simulink model "example1"  (R2024b)
settings: Solver=FixedStepAuto  StartTime=0.0  StopTime=20  FixedStep=0.001  RelTol=1e-3
(part 2 of 3)

== system example1/alpha1 ==
  p/q : Inport
  sumDFj-DFi : Inport  Port=2
  ei1 : Inport  Port=3
  x11 : Inport  Port=4
  Constant : Constant  Value=2
  Gain : Gain  Gain=-1
  Gain1 : Gain  Gain=-0.5
  SAT : Subsystem  Commented=through
  Scope : Scope
  Scope1 : Scope
  Scope2 : Scope
  Sum : Sum  Inputs=|+-
  Sum1 : Sum  Inputs=|++
  Sum2 : Sum  Inputs=|+-
  Sum3 : Sum  Inputs=+++
  "[2]^1_1" : Subsystem
  "[2]^1_2" : Subsystem
  g11 : Subsystem
  alpha1 : Outport
  wires:
  Constant/1 -> Sum/1
  p/q/1 -> "[2]^1_2"/1(p/q), Sum/2
  ei1/1 -> "[2]^1_2"/2(2), "[2]^1_1"/2(2), Gain1/1, Scope/1
  Sum/1 -> "[2]^1_1"/1(In1)
  "[2]^1_1"/1(Out1) -> Sum1/1
  "[2]^1_2"/1(Out1) -> Sum1/2
  Sum1/1 -> Gain/1
  Gain/1 -> Sum3/2
  Sum3/1 -> Sum2/1, Scope2/1
  Gain1/1 -> Sum3/1
  sumDFj-DFi/1 -> Scope1/1, Sum3/3
  g11/1(g11) -> Sum2/2
  x11/1 -> g11/1(x11)
  Sum2/1 -> SAT/1(In1)
  SAT/1(u1) -> alpha1/1

== system example1/alpha2 ==
  p/q : Inport
  sumDFj-DFi : Inport  Port=2
  ei2 : Inport  Port=3
  x21 : Inport  Port=4
  Constant : Constant  Value=2
  Gain : Gain  Gain=-1
  Gain1 : Gain  Gain=-0.5
  Sum : Sum  Inputs=|+-
  Sum1 : Sum  Inputs=|++
  Sum2 : Sum  Inputs=|+-
  Sum3 : Sum  Inputs=+++
  "[2]^1_1" : Subsystem
  "[2]^1_2" : Subsystem
  g21 : Subsystem
  alpha2 : Outport
  wires:
  Constant/1 -> Sum/1
  p/q/1 -> "[2]^1_1"/1(p/q), Sum/2
  ei2/1 -> "[2]^1_1"/2(2), "[2]^1_2"/2(2), Gain1/1
  Sum/1 -> "[2]^1_2"/1(In1)
  "[2]^1_2"/1(Out1) -> Sum1/1
  "[2]^1_1"/1(Out1) -> Sum1/2
  Sum1/1 -> Gain/1
  Gain/1 -> Sum3/2
  Gain1/1 -> Sum3/1
  sumDFj-DFi/1 -> Sum3/3
  Sum3/1 -> Sum2/1
  Sum2/1 -> alpha2/1
  x21/1 -> g21/1(x21)
  g21/1(g21) -> Sum2/2

== system example1/alpha3 ==
  p/q : Inport
  sumDFj-DFi : Inport  Port=2
  ei3 : Inport  Port=3
  x31 : Inport  Port=4
  Constant : Constant  Value=2
  Gain : Gain  Gain=-1
  Gain1 : Gain  Gain=-0.5
  Scope : Scope
  Scope1 : Scope
  Sum : Sum  Inputs=|+-
  Sum1 : Sum  Inputs=|++
  Sum2 : Sum  Inputs=|+-
  Sum3 : Sum  Inputs=+++
  Sum4 : Sum  Inputs=|+-
  "[2]^1_1" : Subsystem
  "[2]^1_2" : Subsystem
  g11 : Subsystem
  alpha3 : Outport
  wires:
  Constant/1 -> Sum/1
  p/q/1 -> Sum/2, "[2]^1_1"/1(p/q)
  ei3/1 -> "[2]^1_1"/2(2), "[2]^1_2"/2(2), Gain1/1
  Sum/1 -> "[2]^1_2"/1(In1)
  "[2]^1_2"/1(Out1) -> Sum1/1
  "[2]^1_1"/1(Out1) -> Sum1/2
  Sum1/1 -> Scope/1, Gain/1
  Gain/1 -> Sum3/2
  Gain1/1 -> Sum3/1
  sumDFj-DFi/1 -> Sum3/3
  Sum3/1 -> Sum2/1
  x31/1 -> g11/1(x11)
  g11/1(g11) -> Scope1/1, Sum2/2
  Sum2/1 -> Sum4/1
  Sum4/1 -> alpha3/1

== system example1/alpha4 ==
  p/q : Inport
  ei4 : Inport  Port=2
  sumDFj-DFi : Inport  Port=3
  x41 : Inport  Port=4
  Constant : Constant  Value=2
  Gain : Gain  Gain=-1
  Gain1 : Gain  Gain=-0.5
  Pow : Math  Operator=pow  SignedPower=on  RndMeth=Zero
  Pow1 : Math  Operator=pow  SignedPower=on  RndMeth=Zero
  Sum : Sum  Inputs=|+-
  Sum1 : Sum  Inputs=|++
  Sum3 : Sum  Inputs=+++
  Sum4 : Sum  Inputs=|+-
  g21 : Subsystem
  alpha4 : Outport
  wires:
  Constant/1 -> Sum/1
  p/q/1 -> Pow1/2, Sum/2
  ei4/1 -> Pow1/1, Gain1/1, Pow/1
  Sum/1 -> Pow/2
  Pow/1 -> Sum1/1
  Pow1/1 -> Sum1/2
  Sum1/1 -> Gain/1
  Gain/1 -> Sum3/2
  Gain1/1 -> Sum3/1
  sumDFj-DFi/1 -> Sum3/3
  Sum3/1 -> Sum4/1
  Sum4/1 -> alpha4/1
  x41/1 -> g21/1(x21)
  g21/1(g21) -> Sum4/2

== system example1/alpha5 ==
  p/q : Inport
  sumDFj-DFi : Inport  Port=2
  ei1 : Inport  Port=3
  x11 : Inport  Port=4
  Constant : Constant  Value=2
  Gain : Gain  Gain=-1
  Gain1 : Gain  Gain=-0.5
  SAT : Subsystem  Commented=through
  Scope : Scope
  Scope1 : Scope
  Scope2 : Scope
  Sum : Sum  Inputs=|+-
  Sum1 : Sum  Inputs=|++
  Sum2 : Sum  Inputs=|+-
  Sum3 : Sum  Inputs=+++
  "[2]^1_1" : Subsystem
  "[2]^1_2" : Subsystem
  g11 : Subsystem
  alpha1 : Outport
  wires:
  Constant/1 -> Sum/1
  p/q/1 -> "[2]^1_2"/1(p/q), Sum/2
  ei1/1 -> "[2]^1_2"/2(2), "[2]^1_1"/2(2), Gain1/1, Scope/1
  Sum/1 -> "[2]^1_1"/1(In1)
  "[2]^1_1"/1(Out1) -> Sum1/1
  "[2]^1_2"/1(Out1) -> Sum1/2
  Sum1/1 -> Gain/1
  Gain/1 -> Sum3/2
  Sum3/1 -> Sum2/1, Scope2/1
  Gain1/1 -> Sum3/1
  sumDFj-DFi/1 -> Scope1/1, Sum3/3
  g11/1(g11) -> Sum2/2
  x11/1 -> g11/1(x11)
  Sum2/1 -> SAT/1(In1)
  SAT/1(u1) -> alpha1/1

== system example1/alpha6 ==
  p/q : Inport
  sumDFj-DFi : Inport  Port=2
  ei2 : Inport  Port=3
  x21 : Inport  Port=4
  Constant : Constant  Value=2
  Gain : Gain  Gain=-1
  Gain1 : Gain  Gain=-0.5
  Sum : Sum  Inputs=|+-
  Sum1 : Sum  Inputs=|++
  Sum2 : Sum  Inputs=|+-
  Sum3 : Sum  Inputs=+++
  "[2]^1_1" : Subsystem
  "[2]^1_2" : Subsystem
  g21 : Subsystem
  alpha2 : Outport
  wires:
  Constant/1 -> Sum/1
  p/q/1 -> "[2]^1_1"/1(p/q), Sum/2
  ei2/1 -> "[2]^1_1"/2(2), "[2]^1_2"/2(2), Gain1/1
  Sum/1 -> "[2]^1_2"/1(In1)
  "[2]^1_2"/1(Out1) -> Sum1/1
  "[2]^1_1"/1(Out1) -> Sum1/2
  Sum1/1 -> Gain/1
  Gain/1 -> Sum3/2
  Gain1/1 -> Sum3/1
  sumDFj-DFi/1 -> Sum3/3
  Sum3/1 -> Sum2/1
  Sum2/1 -> alpha2/1
  x21/1 -> g21/1(x21)
  g21/1(g21) -> Sum2/2

== system example1/alpha7 ==
  p/q : Inport
  sumDFj-DFi : Inport  Port=2
  ei3 : Inport  Port=3
  x31 : Inport  Port=4
  Constant : Constant  Value=2
  Gain : Gain  Gain=-1
  Gain1 : Gain  Gain=-0.5
  Scope : Scope
  Scope1 : Scope
  Sum : Sum  Inputs=|+-
  Sum1 : Sum  Inputs=|++
  Sum2 : Sum  Inputs=|+-
  Sum3 : Sum  Inputs=+++
  Sum4 : Sum  Inputs=|+-
  "[2]^1_1" : Subsystem
  "[2]^1_2" : Subsystem
  g11 : Subsystem
  alpha3 : Outport
  wires:
  Constant/1 -> Sum/1
  p/q/1 -> Sum/2, "[2]^1_1"/1(p/q)
  ei3/1 -> "[2]^1_1"/2(2), "[2]^1_2"/2(2), Gain1/1
  Sum/1 -> "[2]^1_2"/1(In1)
  "[2]^1_2"/1(Out1) -> Sum1/1
  "[2]^1_1"/1(Out1) -> Sum1/2
  Sum1/1 -> Scope/1, Gain/1
  Gain/1 -> Sum3/2
  Gain1/1 -> Sum3/1
  sumDFj-DFi/1 -> Sum3/3
  Sum3/1 -> Sum2/1
  x31/1 -> g11/1(x11)
  g11/1(g11) -> Scope1/1, Sum2/2
  Sum2/1 -> Sum4/1
  Sum4/1 -> alpha3/1

== system example1/alpha8 ==
  p/q : Inport
  ei4 : Inport  Port=2
  sumDFj-DFi : Inport  Port=3
  x41 : Inport  Port=4
  Constant : Constant  Value=2
  Gain : Gain  Gain=-1
  Gain1 : Gain  Gain=-0.5
  Pow : Math  Operator=pow  SignedPower=on  RndMeth=Zero
  Pow1 : Math  Operator=pow  SignedPower=on  RndMeth=Zero
  Sum : Sum  Inputs=|+-
  Sum1 : Sum  Inputs=|++
  Sum3 : Sum  Inputs=+++
  Sum4 : Sum  Inputs=|+-
  g21 : Subsystem
  alpha4 : Outport
  wires:
  Constant/1 -> Sum/1
  p/q/1 -> Pow1/2, Sum/2
  ei4/1 -> Pow1/1, Gain1/1, Pow/1
  Sum/1 -> Pow/2
  Pow/1 -> Sum1/1
  Pow1/1 -> Sum1/2
  Sum1/1 -> Gain/1
  Gain/1 -> Sum3/2
  Gain1/1 -> Sum3/1
  sumDFj-DFi/1 -> Sum3/3
  Sum3/1 -> Sum4/1
  Sum4/1 -> alpha4/1
  x41/1 -> g21/1(x21)
  g21/1(g21) -> Sum4/2

== system example1/j-i_1 ==
  DFi : Inport
  DFi+1 : Inport  Port=2
  DFi-1 : Inport  Port=3
  p/q : Inport  Port=4
  Add : Sum  Inputs=+-
  Add1 : Sum  Inputs=-+
  Add2 : Sum  Inputs=-+
  Sum : Sum  Inputs=|++
  Sum1 : Sum  Inputs=|++
  Sum2 : Sum  Inputs=|++
  "[2]^1_1" : Subsystem
  "[2]^1_2" : Subsystem
  "[2]^1_3" : Subsystem
  "[2]^1_4" : Subsystem
  constant : Constant  Value=2
  j-i : Outport
  wires:
  DFi-1/1 -> Add/1
  DFi/1 -> Add1/1, Add/2
  DFi+1/1 -> Add1/2
  p/q/1 -> "[2]^1_4"/1(In1), "[2]^1_3"/1(p/q), Add2/1
  constant/1 -> Add2/2
  Add/1 -> "[2]^1_3"/2(2), "[2]^1_1"/2(2)
  Add2/1 -> "[2]^1_2"/1(In1), "[2]^1_1"/1(In1)
  Add1/1 -> "[2]^1_4"/2(2), "[2]^1_2"/2(2)
  "[2]^1_1"/1(Out1) -> Sum/1
  "[2]^1_2"/1(Out1) -> Sum/2
  "[2]^1_3"/1(Out1) -> Sum1/1
  "[2]^1_4"/1(Out1) -> Sum1/2
  Sum/1 -> Sum2/1
  Sum1/1 -> Sum2/2
  Sum2/1 -> j-i/1

== system example1/j-i_2 ==
  DFi : Inport
  DFi+1 : Inport  Port=2
  DFi-1 : Inport  Port=3
  p/q : Inport  Port=4
  Add : Sum  Inputs=+-
  Add1 : Sum  Inputs=-+
  Add2 : Sum  Inputs=-+
  Sum : Sum  Inputs=|++
  Sum1 : Sum  Inputs=|++
  Sum2 : Sum  Inputs=|++
  "[2]^1_1" : Subsystem
  "[2]^1_2" : Subsystem
  "[2]^1_3" : Subsystem
  "[2]^1_4" : Subsystem
  constant : Constant  Value=2
  j-i : Outport
  wires:
  DFi-1/1 -> Add/1
  DFi/1 -> Add1/1, Add/2
  DFi+1/1 -> Add1/2
  p/q/1 -> "[2]^1_4"/1(In1), "[2]^1_3"/1(In1), Add2/1
  constant/1 -> Add2/2
  Add/1 -> "[2]^1_3"/2(2), "[2]^1_1"/2(2)
  Add2/1 -> "[2]^1_2"/1(In1), "[2]^1_1"/1(In1)
  Add1/1 -> "[2]^1_4"/2(2), "[2]^1_2"/2(2)
  "[2]^1_1"/1(Out1) -> Sum/1
  "[2]^1_2"/1(Out1) -> Sum/2
  "[2]^1_3"/1(Out1) -> Sum1/1
  "[2]^1_4"/1(Out1) -> Sum1/2
  Sum/1 -> Sum2/1
  Sum1/1 -> Sum2/2
  Sum2/1 -> j-i/1

== system example1/j-i_3 ==
  DFi : Inport
  DFi+1 : Inport  Port=2
  DFi-1 : Inport  Port=3
  p/q : Inport  Port=4
  Add : Sum  Inputs=+-
  Add1 : Sum  Inputs=-+
  Add2 : Sum  Inputs=-+
  Pow{,1..3} (4 alike) : Math  Operator=pow  SignedPower=on  RndMeth=Zero
  Scope : Scope
  Scope1 : Scope
  Sum : Sum  Inputs=|++
  Sum1 : Sum  Inputs=|++
  Sum2 : Sum  Inputs=|++
  constant : Constant  Value=2
  j-i : Outport
  wires:
  DFi-1/1 -> Add/1
  DFi/1 -> Add1/1, Add/2
  DFi+1/1 -> Add1/2
  p/q/1 -> Pow3/2, Pow2/2, Add2/1
  constant/1 -> Add2/2
  Add/1 -> Scope1/1, Pow/1, Pow2/1
  Add2/1 -> Pow1/2, Pow/2
  Add1/1 -> Pow3/1, Pow1/1
  Pow/1 -> Sum/1
  Pow1/1 -> Sum/2
  Pow2/1 -> Sum1/1
  Pow3/1 -> Sum1/2
  Sum/1 -> Scope/1, Sum2/1
  Sum1/1 -> Sum2/2
  Sum2/1 -> j-i/1

== system example1/j-i_4 ==
  DFi : Inport
  DFi+1 : Inport  Port=2
  DFi-1 : Inport  Port=3
  p/q : Inport  Port=4
  Add : Sum  Inputs=+-
  Add1 : Sum  Inputs=-+
  Add2 : Sum  Inputs=-+
  Pow{,1..3} (4 alike) : Math  Operator=pow  SignedPower=on  RndMeth=Zero
  Sum : Sum  Inputs=|++
  Sum1 : Sum  Inputs=|++
  Sum2 : Sum  Inputs=|++
  constant : Constant  Value=2
  j-i : Outport
  wires:
  DFi-1/1 -> Add/1
  DFi/1 -> Add1/1, Add/2
  DFi+1/1 -> Add1/2
  p/q/1 -> Pow3/2, Pow2/2, Add2/1
  constant/1 -> Add2/2
  Add/1 -> Pow2/1, Pow/1
  Add2/1 -> Pow1/2, Pow/2
  Add1/1 -> Pow3/1, Pow1/1
  Pow/1 -> Sum/1
  Pow1/1 -> Sum/2
  Pow2/1 -> Sum1/1
  Pow3/1 -> Sum1/2
  Sum/1 -> Sum2/1
  Sum1/1 -> Sum2/2
  Sum2/1 -> j-i/1

== system example1/j-i_5 ==
  DFi : Inport
  DFi+1 : Inport  Port=2
  DFi-1 : Inport  Port=3
  p/q : Inport  Port=4
  Add : Sum  Inputs=+-
  Add1 : Sum  Inputs=-+
  Add2 : Sum  Inputs=-+
  Gain : Gain
  Sum : Sum  Inputs=|++
  Sum1 : Sum  Inputs=|++
  Sum2 : Sum  Inputs=|++
  "[2]^1_1" : Subsystem
  "[2]^1_2" : Subsystem
  "[2]^1_3" : Subsystem
  "[2]^1_4" : Subsystem
  constant : Constant  Value=2
  j-i : Outport
  wires:
  DFi-1/1 -> Add/1
  DFi/1 -> Add1/1, Add/2
  DFi+1/1 -> Add1/2
  p/q/1 -> "[2]^1_4"/1(In1), "[2]^1_3"/1(p/q), Add2/1
  constant/1 -> Add2/2
  Add/1 -> "[2]^1_3"/2(2), "[2]^1_1"/2(2)
  Add2/1 -> "[2]^1_2"/1(In1), "[2]^1_1"/1(In1)
  Add1/1 -> "[2]^1_4"/2(2), "[2]^1_2"/2(2)
  "[2]^1_1"/1(Out1) -> Sum/1
  "[2]^1_2"/1(Out1) -> Sum/2
  "[2]^1_3"/1(Out1) -> Sum1/1
  "[2]^1_4"/1(Out1) -> Sum1/2
  Sum/1 -> Sum2/1
  Sum1/1 -> Sum2/2
  Sum2/1 -> Gain/1
  Gain/1 -> j-i/1

== system example1/j-i_6 ==
  DFi : Inport
  DFi+1 : Inport  Port=2
  DFi-1 : Inport  Port=3
  p/q : Inport  Port=4
  Add : Sum  Inputs=+-
  Add1 : Sum  Inputs=-+
  Add2 : Sum  Inputs=-+
  Gain : Gain
  Sum : Sum  Inputs=|++
  Sum1 : Sum  Inputs=|++
  Sum2 : Sum  Inputs=|++
  "[2]^1_1" : Subsystem
  "[2]^1_2" : Subsystem
  "[2]^1_3" : Subsystem
  "[2]^1_4" : Subsystem
  constant : Constant  Value=2
  j-i : Outport
  wires:
  DFi-1/1 -> Add/1
  DFi/1 -> Add1/1, Add/2
  DFi+1/1 -> Add1/2
  p/q/1 -> "[2]^1_4"/1(In1), "[2]^1_3"/1(In1), Add2/1
  constant/1 -> Add2/2
  Add/1 -> "[2]^1_3"/2(2), "[2]^1_1"/2(2)
  Add2/1 -> "[2]^1_2"/1(In1), "[2]^1_1"/1(In1)
  Add1/1 -> "[2]^1_4"/2(2), "[2]^1_2"/2(2)
  "[2]^1_1"/1(Out1) -> Sum/1
  "[2]^1_2"/1(Out1) -> Sum/2
  "[2]^1_3"/1(Out1) -> Sum1/1
  "[2]^1_4"/1(Out1) -> Sum1/2
  Sum/1 -> Sum2/1
  Sum1/1 -> Sum2/2
  Gain/1 -> j-i/1
  Sum2/1 -> Gain/1

== system example1/j-i_7 ==
  DFi : Inport
  DFi+1 : Inport  Port=2
  DFi-1 : Inport  Port=3
  p/q : Inport  Port=4
  Add : Sum  Inputs=+-
  Add1 : Sum  Inputs=-+
  Add2 : Sum  Inputs=-+
  Gain : Gain
  Pow{,1..3} (4 alike) : Math  Operator=pow  SignedPower=on  RndMeth=Zero
  Scope : Scope
  Scope1 : Scope
  Sum : Sum  Inputs=|++
  Sum1 : Sum  Inputs=|++
  Sum2 : Sum  Inputs=|++
  constant : Constant  Value=2
  j-i : Outport
  wires:
  DFi-1/1 -> Add/1
  DFi/1 -> Add1/1, Add/2
  DFi+1/1 -> Add1/2
  p/q/1 -> Pow3/2, Pow2/2, Add2/1
  constant/1 -> Add2/2
  Add/1 -> Scope1/1, Pow/1, Pow2/1
  Add2/1 -> Pow1/2, Pow/2
  Add1/1 -> Pow3/1, Pow1/1
  Pow/1 -> Sum/1
  Pow1/1 -> Sum/2
  Pow2/1 -> Sum1/1
  Pow3/1 -> Sum1/2
  Sum/1 -> Scope/1, Sum2/1
  Sum1/1 -> Sum2/2
  Sum2/1 -> Gain/1
  Gain/1 -> j-i/1

== system example1/j-i_8 ==
  DFi : Inport
  DFi+1 : Inport  Port=2
  DFi-1 : Inport  Port=3
  p/q : Inport  Port=4
  Add : Sum  Inputs=+-
  Add1 : Sum  Inputs=-+
  Add2 : Sum  Inputs=-+
  Gain : Gain
  Pow{,1..3} (4 alike) : Math  Operator=pow  SignedPower=on  RndMeth=Zero
  Sum : Sum  Inputs=|++
  Sum1 : Sum  Inputs=|++
  Sum2 : Sum  Inputs=|++
  constant : Constant  Value=2
  j-i : Outport
  wires:
  DFi-1/1 -> Add/1
  DFi/1 -> Add1/1, Add/2
  DFi+1/1 -> Add1/2
  p/q/1 -> Pow3/2, Pow2/2, Add2/1
  constant/1 -> Add2/2
  Add/1 -> Pow2/1, Pow/1
  Add2/1 -> Pow1/2, Pow/2
  Add1/1 -> Pow3/1, Pow1/1
  Pow/1 -> Sum/1
  Pow1/1 -> Sum/2
  Pow2/1 -> Sum1/1
  Pow3/1 -> Sum1/2
  Sum/1 -> Sum2/1
  Sum1/1 -> Sum2/2
  Sum2/1 -> Gain/1
  Gain/1 -> j-i/1

== system example1/ESTIMAT1/[2]^1 ==
  In1 : Inport
  In2 : Inport  Port=2
  Abs : Abs  SaturateOnIntegerOverflow=off
  Pow : Math  Operator=pow  SignedPower=on  RndMeth=Zero
  Product : Product
  Sign : Signum
  Out1 : Outport
  wires:
  Pow/1 -> Product/1
  In2/1 -> Abs/1, Sign/1
  Abs/1 -> Pow/1
  Sign/1 -> Product/2
  Product/1 -> Out1/1
  In1/1 -> Pow/2

== system example1/ESTIMAT1/[2]^2 ==
  beta1 : Inport
  In2 : Inport  Port=2
  Abs : Abs  SaturateOnIntegerOverflow=off
  Pow : Math  Operator=pow  SignedPower=on  RndMeth=Zero
  Product : Product
  Sign : Signum
  Out1 : Outport
  wires:
  Pow/1 -> Product/1
  In2/1 -> Abs/1, Sign/1
  Abs/1 -> Pow/1
  Sign/1 -> Product/2
  Product/1 -> Out1/1
  beta1/1 -> Pow/2

== system example1/ESTIMAT1/[2]^3 ==
  In1 : Inport
  In2 : Inport  Port=2
  Abs : Abs  SaturateOnIntegerOverflow=off
  Pow : Math  Operator=pow  SignedPower=on  RndMeth=Zero
  Product : Product
  Sign : Signum
  Out1 : Outport
  wires:
  Pow/1 -> Product/1
  In2/1 -> Abs/1, Sign/1
  Abs/1 -> Pow/1
  Sign/1 -> Product/2
  Product/1 -> Out1/1
  In1/1 -> Pow/2

== system example1/ESTIMAT1/[2]^4 ==
  beta1 : Inport
  In2 : Inport  Port=2
  Abs : Abs  SaturateOnIntegerOverflow=off
  Pow : Math  Operator=pow  SignedPower=on  RndMeth=Zero
  Product : Product
  Sign : Signum
  Out1 : Outport
  wires:
  Pow/1 -> Product/1
  In2/1 -> Abs/1, Sign/1
  Abs/1 -> Pow/1
  Sign/1 -> Product/2
  Product/1 -> Out1/1
  beta1/1 -> Pow/2

== system example1/ESTIMAT1/[2]^5 ==
  In1 : Inport
  In2 : Inport  Port=2
  Abs : Abs  SaturateOnIntegerOverflow=off
  Pow : Math  Operator=pow  SignedPower=on  RndMeth=Zero
  Product : Product
  Sign : Signum
  Out1 : Outport
  wires:
  Pow/1 -> Product/1
  In2/1 -> Abs/1, Sign/1
  Abs/1 -> Pow/1
  Sign/1 -> Product/2
  Product/1 -> Out1/1
  In1/1 -> Pow/2

== system example1/ESTIMAT1/[2]^6 ==
  beta1 : Inport
  In2 : Inport  Port=2
  Abs : Abs  SaturateOnIntegerOverflow=off
  Pow : Math  Operator=pow  SignedPower=on  RndMeth=Zero
  Product : Product
  Sign : Signum
  Out1 : Outport
  wires:
  Pow/1 -> Product/1
  In2/1 -> Abs/1, Sign/1
  Abs/1 -> Pow/1
  Sign/1 -> Product/2
  Product/1 -> Out1/1
  beta1/1 -> Pow/2

== system example1/ESTIMAT1/g11 ==
  x11 : Inport
  Cos : Trigonometry  Operator=cos
  Sum : Sum  Inputs=|++
  g11 : Outport
  wires:
  Cos/1 -> Sum/1
  Sum/1 -> g11/1
  x11/1 -> Sum/2, Cos/1

== system example1/ESTIMAT1/g12 ==
  x11 : Inport
  x12 : Inport  Port=2
  Cos : Trigonometry  Operator=cos
  Sin : Trigonometry
  Sum : Sum  Inputs=|++
  g12 : Outport
  wires:
  x12/1 -> Sin/1
  x11/1 -> Cos/1
  Cos/1 -> Sum/1
  Sin/1 -> Sum/2
  Sum/1 -> g12/1

== system example1/ESTIMAT2/[2]^1 ==
  In1 : Inport
  In2 : Inport  Port=2
  Abs : Abs  SaturateOnIntegerOverflow=off
  Pow : Math  Operator=pow  SignedPower=on  RndMeth=Zero
  Product : Product
  Sign : Signum
  Out1 : Outport
  wires:
  Pow/1 -> Product/1
  In2/1 -> Abs/1, Sign/1
  Abs/1 -> Pow/1
  Sign/1 -> Product/2
  Product/1 -> Out1/1
  In1/1 -> Pow/2

== system example1/ESTIMAT2/[2]^2 ==
  beta1 : Inport
  In2 : Inport  Port=2
  Abs : Abs  SaturateOnIntegerOverflow=off
  Pow : Math  Operator=pow  SignedPower=on  RndMeth=Zero
  Product : Product
  Sign : Signum
  Out1 : Outport
  wires:
  Pow/1 -> Product/1
  In2/1 -> Abs/1, Sign/1
  Abs/1 -> Pow/1
  Sign/1 -> Product/2
  Product/1 -> Out1/1
  beta1/1 -> Pow/2

== system example1/ESTIMAT2/[2]^3 ==
  In1 : Inport
  In2 : Inport  Port=2
  Abs : Abs  SaturateOnIntegerOverflow=off
  Pow : Math  Operator=pow  SignedPower=on  RndMeth=Zero
  Product : Product
  Sign : Signum
  Out1 : Outport
  wires:
  Pow/1 -> Product/1
  In2/1 -> Abs/1, Sign/1
  Abs/1 -> Pow/1
  Sign/1 -> Product/2
  Product/1 -> Out1/1
  In1/1 -> Pow/2

== system example1/ESTIMAT2/[2]^4 ==
  beta1 : Inport
  In2 : Inport  Port=2
  Abs : Abs  SaturateOnIntegerOverflow=off
  Pow : Math  Operator=pow  SignedPower=on  RndMeth=Zero
  Product : Product
  Sign : Signum
  Out1 : Outport
  wires:
  Pow/1 -> Product/1
  In2/1 -> Abs/1, Sign/1
  Abs/1 -> Pow/1
  Sign/1 -> Product/2
  Product/1 -> Out1/1
  beta1/1 -> Pow/2

== system example1/ESTIMAT2/[2]^5 ==
  In1 : Inport
  In2 : Inport  Port=2
  Abs : Abs  SaturateOnIntegerOverflow=off
  Pow : Math  Operator=pow  SignedPower=on  RndMeth=Zero
  Product : Product
  Sign : Signum
  Out1 : Outport
  wires:
  Pow/1 -> Product/1
  In2/1 -> Abs/1, Sign/1
  Abs/1 -> Pow/1
  Sign/1 -> Product/2
  Product/1 -> Out1/1
  In1/1 -> Pow/2

== system example1/ESTIMAT2/[2]^6 ==
  beta1 : Inport
  In2 : Inport  Port=2
  Abs : Abs  SaturateOnIntegerOverflow=off
  Pow : Math  Operator=pow  SignedPower=on  RndMeth=Zero
  Product : Product
  Sign : Signum
  Out1 : Outport
  wires:
  Pow/1 -> Product/1
  In2/1 -> Abs/1, Sign/1
  Abs/1 -> Pow/1
  Sign/1 -> Product/2
  Product/1 -> Out1/1
  beta1/1 -> Pow/2

== system example1/ESTIMAT2/g21 ==
  x21 : Inport
  Cos : Trigonometry  Operator=cos
  Product : Product
  Sin : Trigonometry
  Sum : Sum  Inputs=|++
  g21 : Outport
  wires:
  x21/1 -> Cos/1, Sin/1, Sum/1
  Sum/1 -> g21/1
  Sin/1 -> Product/1
  Cos/1 -> Product/2
  Product/1 -> Sum/2

== system example1/ESTIMAT2/g22 ==
  x21 : Inport
  x22 : Inport  Port=2
  Sin : Trigonometry
  Sum : Sum  Inputs=|++
  Sum1 : Sum  Inputs=|++
  g22 : Outport
  wires:
  x22/1 -> Sum/2, Sum1/2
  Sum/1 -> g22/1
  x21/1 -> Sum1/1
  Sum1/1 -> Sin/1
  Sin/1 -> Sum/1

== system example1/ESTIMAT3/[2]^1 ==
  In1 : Inport
  In2 : Inport  Port=2
  Abs : Abs  SaturateOnIntegerOverflow=off
  Pow : Math  Operator=pow  SignedPower=on  RndMeth=Zero
  Product : Product
  Sign : Signum
  Out1 : Outport
  wires:
  Pow/1 -> Product/1
  In2/1 -> Abs/1, Sign/1
  Abs/1 -> Pow/1
  Sign/1 -> Product/2
  Product/1 -> Out1/1
  In1/1 -> Pow/2

== system example1/ESTIMAT3/[2]^2 ==
  beta1 : Inport
  In2 : Inport  Port=2
  Abs : Abs  SaturateOnIntegerOverflow=off
  Pow : Math  Operator=pow  SignedPower=on  RndMeth=Zero
  Product : Product
  Sign : Signum
  Out1 : Outport
  wires:
  Pow/1 -> Product/1
  In2/1 -> Abs/1, Sign/1
  Abs/1 -> Pow/1
  Sign/1 -> Product/2
  Product/1 -> Out1/1
  beta1/1 -> Pow/2

== system example1/ESTIMAT3/[2]^3 ==
  In1 : Inport
  In2 : Inport  Port=2
  Abs : Abs  SaturateOnIntegerOverflow=off
  Pow : Math  Operator=pow  SignedPower=on  RndMeth=Zero
  Product : Product
  Sign : Signum
  Out1 : Outport
  wires:
  Pow/1 -> Product/1
  In2/1 -> Abs/1, Sign/1
  Abs/1 -> Pow/1
  Sign/1 -> Product/2
  Product/1 -> Out1/1
  In1/1 -> Pow/2

== system example1/ESTIMAT3/[2]^4 ==
  beta1 : Inport
  In2 : Inport  Port=2
  Abs : Abs  SaturateOnIntegerOverflow=off
  Pow : Math  Operator=pow  SignedPower=on  RndMeth=Zero
  Product : Product
  Sign : Signum
  Out1 : Outport
  wires:
  Pow/1 -> Product/1
  In2/1 -> Abs/1, Sign/1
  Abs/1 -> Pow/1
  Sign/1 -> Product/2
  Product/1 -> Out1/1
  beta1/1 -> Pow/2

== system example1/ESTIMAT3/[2]^5 ==
  In1 : Inport
  In2 : Inport  Port=2
  Abs : Abs  SaturateOnIntegerOverflow=off
  Pow : Math  Operator=pow  SignedPower=on  RndMeth=Zero
  Product : Product
  Sign : Signum
  Out1 : Outport
  wires:
  Pow/1 -> Product/1
  In2/1 -> Abs/1, Sign/1
  Abs/1 -> Pow/1
  Sign/1 -> Product/2
  Product/1 -> Out1/1
  In1/1 -> Pow/2

== system example1/ESTIMAT3/[2]^6 ==
  beta1 : Inport
  In2 : Inport  Port=2
  Abs : Abs  SaturateOnIntegerOverflow=off
  Pow : Math  Operator=pow  SignedPower=on  RndMeth=Zero
  Product : Product
  Sign : Signum
  Out1 : Outport
  wires:
  Pow/1 -> Product/1
  In2/1 -> Abs/1, Sign/1
  Abs/1 -> Pow/1
  Sign/1 -> Product/2
  Product/1 -> Out1/1
  beta1/1 -> Pow/2

== system example1/ESTIMAT3/g11 ==
  x11 : Inport
  Sin : Trigonometry
  g11 : Outport
  wires:
  Sin/1 -> g11/1
  x11/1 -> Sin/1

== system example1/ESTIMAT3/g12 ==
  x11 : Inport
  x12 : Inport  Port=2
  Add : Sum  Inputs=3
  Cos : Trigonometry  Operator=cos
  Product : Product
  Sin : Trigonometry
  Sin1 : Trigonometry
  g12 : Outport
  wires:
  x12/1 -> Product/2, Sin/1
  Sin/1 -> Add/2
  Add/1 -> g12/1
  x11/1 -> Product/1, Cos/1
  Cos/1 -> Add/1
  Product/1 -> Sin1/1

== system example1/ESTIMAT4/[2]^1 ==
  In1 : Inport
  In2 : Inport  Port=2
  Abs : Abs  SaturateOnIntegerOverflow=off
  Pow : Math  Operator=pow  SignedPower=on  RndMeth=Zero
  Product : Product
  Sign : Signum
  Out1 : Outport
  wires:
  Pow/1 -> Product/1
  In2/1 -> Abs/1, Sign/1
  Abs/1 -> Pow/1
  Sign/1 -> Product/2
  Product/1 -> Out1/1
  In1/1 -> Pow/2

== system example1/ESTIMAT4/[2]^2 ==
  beta1 : Inport
  In2 : Inport  Port=2
  Abs : Abs  SaturateOnIntegerOverflow=off
  Pow : Math  Operator=pow  SignedPower=on  RndMeth=Zero
  Product : Product
  Sign : Signum
  Out1 : Outport
  wires:
  Pow/1 -> Product/1
  In2/1 -> Abs/1, Sign/1
  Abs/1 -> Pow/1
  Sign/1 -> Product/2
  Product/1 -> Out1/1
  beta1/1 -> Pow/2

== system example1/ESTIMAT4/[2]^3 ==
  In1 : Inport
  In2 : Inport  Port=2
  Abs : Abs  SaturateOnIntegerOverflow=off
  Pow : Math  Operator=pow  SignedPower=on  RndMeth=Zero
  Product : Product
  Sign : Signum
  Out1 : Outport
  wires:
  Pow/1 -> Product/1
  In2/1 -> Abs/1, Sign/1
  Abs/1 -> Pow/1
  Sign/1 -> Product/2
  Product/1 -> Out1/1
  In1/1 -> Pow/2

== system example1/ESTIMAT4/[2]^4 ==
  beta1 : Inport
  In2 : Inport  Port=2
  Abs : Abs  SaturateOnIntegerOverflow=off
  Pow : Math  Operator=pow  SignedPower=on  RndMeth=Zero
  Product : Product
  Sign : Signum
  Out1 : Outport
  wires:
  Pow/1 -> Product/1
  In2/1 -> Abs/1, Sign/1
  Abs/1 -> Pow/1
  Sign/1 -> Product/2
  Product/1 -> Out1/1
  beta1/1 -> Pow/2

== system example1/ESTIMAT4/[2]^5 ==
  In1 : Inport
  In2 : Inport  Port=2
  Abs : Abs  SaturateOnIntegerOverflow=off
  Pow : Math  Operator=pow  SignedPower=on  RndMeth=Zero
  Product : Product
  Sign : Signum
  Out1 : Outport
  wires:
  Pow/1 -> Product/1
  In2/1 -> Abs/1, Sign/1
  Abs/1 -> Pow/1
  Sign/1 -> Product/2
  Product/1 -> Out1/1
  In1/1 -> Pow/2

== system example1/ESTIMAT4/[2]^6 ==
  beta1 : Inport
  In2 : Inport  Port=2
  Abs : Abs  SaturateOnIntegerOverflow=off
  Pow : Math  Operator=pow  SignedPower=on  RndMeth=Zero
  Product : Product
  Sign : Signum
  Out1 : Outport
  wires:
  Pow/1 -> Product/1
  In2/1 -> Abs/1, Sign/1
  Abs/1 -> Pow/1
  Sign/1 -> Product/2
  Product/1 -> Out1/1
  beta1/1 -> Pow/2

== system example1/ESTIMAT4/g21 ==
  x21 : Inport
  Cos : Trigonometry  Operator=cos
  Product : Product
  Product1 : Product
  Sin : Trigonometry
  g21 : Outport
  wires:
  x21/1 -> Cos/1, Sin/1
  Sin/1 -> Product/1
  Product/1 -> g21/1
  Cos/1 -> Product1/1, Product1/2
  Product1/1 -> Product/2

== system example1/ESTIMAT4/g22 ==
  x21 : Inport
  x22 : Inport  Port=2
  Constant : Constant  Value=4/5
  Sin : Trigonometry
  Sum : Sum  Inputs=|++
  Sum1 : Sum  Inputs=|++
  "[2]^1_1" : Subsystem
  g22 : Outport
  wires:
  x22/1 -> Sum1/2, "[2]^1_1"/2(2)
  Constant/1 -> "[2]^1_1"/1(In1)
  "[2]^1_1"/1(Out1) -> Sum/2
  Sum/1 -> g22/1
  x21/1 -> Sum1/1
  Sum1/1 -> Sin/1
  Sin/1 -> Sum/1

== system example1/ESTIMAT5/[2]^1 ==
  In1 : Inport
  In2 : Inport  Port=2
  Abs : Abs  SaturateOnIntegerOverflow=off
  Pow : Math  Operator=pow  SignedPower=on  RndMeth=Zero
  Product : Product
  Sign : Signum
  Out1 : Outport
  wires:
  Pow/1 -> Product/1
  In2/1 -> Abs/1, Sign/1
  Abs/1 -> Pow/1
  Sign/1 -> Product/2
  Product/1 -> Out1/1
  In1/1 -> Pow/2

== system example1/ESTIMAT5/[2]^2 ==
  beta1 : Inport
  In2 : Inport  Port=2
  Abs : Abs  SaturateOnIntegerOverflow=off
  Pow : Math  Operator=pow  SignedPower=on  RndMeth=Zero
  Product : Product
  Sign : Signum
  Out1 : Outport
  wires:
  Pow/1 -> Product/1
  In2/1 -> Abs/1, Sign/1
  Abs/1 -> Pow/1
  Sign/1 -> Product/2
  Product/1 -> Out1/1
  beta1/1 -> Pow/2

== system example1/ESTIMAT5/[2]^3 ==
  In1 : Inport
  In2 : Inport  Port=2
  Abs : Abs  SaturateOnIntegerOverflow=off
  Pow : Math  Operator=pow  SignedPower=on  RndMeth=Zero
  Product : Product
  Sign : Signum
  Out1 : Outport
  wires:
  Pow/1 -> Product/1
  In2/1 -> Abs/1, Sign/1
  Abs/1 -> Pow/1
  Sign/1 -> Product/2
  Product/1 -> Out1/1
  In1/1 -> Pow/2

== system example1/ESTIMAT5/[2]^4 ==
  beta1 : Inport
  In2 : Inport  Port=2
  Abs : Abs  SaturateOnIntegerOverflow=off
  Pow : Math  Operator=pow  SignedPower=on  RndMeth=Zero
  Product : Product
  Sign : Signum
  Out1 : Outport
  wires:
  Pow/1 -> Product/1
  In2/1 -> Abs/1, Sign/1
  Abs/1 -> Pow/1
  Sign/1 -> Product/2
  Product/1 -> Out1/1
  beta1/1 -> Pow/2

== system example1/ESTIMAT5/[2]^5 ==
  In1 : Inport
  In2 : Inport  Port=2
  Abs : Abs  SaturateOnIntegerOverflow=off
  Pow : Math  Operator=pow  SignedPower=on  RndMeth=Zero
  Product : Product
  Sign : Signum
  Out1 : Outport
  wires:
  Pow/1 -> Product/1
  In2/1 -> Abs/1, Sign/1
  Abs/1 -> Pow/1
  Sign/1 -> Product/2
  Product/1 -> Out1/1
  In1/1 -> Pow/2

== system example1/ESTIMAT5/[2]^6 ==
  beta1 : Inport
  In2 : Inport  Port=2
  Abs : Abs  SaturateOnIntegerOverflow=off
  Pow : Math  Operator=pow  SignedPower=on  RndMeth=Zero
  Product : Product
  Sign : Signum
  Out1 : Outport
  wires:
  Pow/1 -> Product/1
  In2/1 -> Abs/1, Sign/1
  Abs/1 -> Pow/1
  Sign/1 -> Product/2
  Product/1 -> Out1/1
  beta1/1 -> Pow/2

== system example1/ESTIMAT5/g21 ==
  x21 : Inport
  Cos : Trigonometry  Operator=cos
  Product : Product
  Sin : Trigonometry  Operator=cos
  Sum : Sum  Inputs=|++
  g21 : Outport
  wires:
  x21/1 -> Sum/1, Sin/1, Cos/1
  Sum/1 -> g21/1
  Sin/1 -> Product/1
  Cos/1 -> Product/2
  Product/1 -> Sum/2

== system example1/ESTIMAT5/g22 ==
  x21 : Inport
  x22 : Inport  Port=2
  Gain : Gain  Gain=-2
  Sin : Trigonometry
  Sum : Sum  Inputs=|++
  Sum1 : Sum  Inputs=|++
  g22 : Outport
  wires:
  x22/1 -> Sum/2, Sum1/2
  Sum/1 -> g22/1
  x21/1 -> Gain/1
  Sum1/1 -> Sin/1
  Sin/1 -> Sum/1
  Gain/1 -> Sum1/1

== system example1/ESTIMAT6/[2]^1 ==
  In1 : Inport
  In2 : Inport  Port=2
  Abs : Abs  SaturateOnIntegerOverflow=off
  Pow : Math  Operator=pow  SignedPower=on  RndMeth=Zero
  Product : Product
  Sign : Signum
  Out1 : Outport
  wires:
  Pow/1 -> Product/1
  In2/1 -> Abs/1, Sign/1
  Abs/1 -> Pow/1
  Sign/1 -> Product/2
  Product/1 -> Out1/1
  In1/1 -> Pow/2

== system example1/ESTIMAT6/[2]^2 ==
  beta1 : Inport
  In2 : Inport  Port=2
  Abs : Abs  SaturateOnIntegerOverflow=off
  Pow : Math  Operator=pow  SignedPower=on  RndMeth=Zero
  Product : Product
  Sign : Signum
  Out1 : Outport
  wires:
  Pow/1 -> Product/1
  In2/1 -> Abs/1, Sign/1
  Abs/1 -> Pow/1
  Sign/1 -> Product/2
  Product/1 -> Out1/1
  beta1/1 -> Pow/2

== system example1/ESTIMAT6/[2]^3 ==
  In1 : Inport
  In2 : Inport  Port=2
  Abs : Abs  SaturateOnIntegerOverflow=off
  Pow : Math  Operator=pow  SignedPower=on  RndMeth=Zero
  Product : Product
  Sign : Signum
  Out1 : Outport
  wires:
  Pow/1 -> Product/1
  In2/1 -> Abs/1, Sign/1
  Abs/1 -> Pow/1
  Sign/1 -> Product/2
  Product/1 -> Out1/1
  In1/1 -> Pow/2

== system example1/ESTIMAT6/[2]^4 ==
  beta1 : Inport
  In2 : Inport  Port=2
  Abs : Abs  SaturateOnIntegerOverflow=off
  Pow : Math  Operator=pow  SignedPower=on  RndMeth=Zero
  Product : Product
  Sign : Signum
  Out1 : Outport
  wires:
  Pow/1 -> Product/1
  In2/1 -> Abs/1, Sign/1
  Abs/1 -> Pow/1
  Sign/1 -> Product/2
  Product/1 -> Out1/1
  beta1/1 -> Pow/2

== system example1/ESTIMAT6/[2]^5 ==
  In1 : Inport
  In2 : Inport  Port=2
  Abs : Abs  SaturateOnIntegerOverflow=off
  Pow : Math  Operator=pow  SignedPower=on  RndMeth=Zero
  Product : Product
  Sign : Signum
  Out1 : Outport
  wires:
  Pow/1 -> Product/1
  In2/1 -> Abs/1, Sign/1
  Abs/1 -> Pow/1
  Sign/1 -> Product/2
  Product/1 -> Out1/1
  In1/1 -> Pow/2

== system example1/ESTIMAT6/[2]^6 ==
  beta1 : Inport
  In2 : Inport  Port=2
  Abs : Abs  SaturateOnIntegerOverflow=off
  Pow : Math  Operator=pow  SignedPower=on  RndMeth=Zero
  Product : Product
  Sign : Signum
  Out1 : Outport
  wires:
  Pow/1 -> Product/1
  In2/1 -> Abs/1, Sign/1
  Abs/1 -> Pow/1
  Sign/1 -> Product/2
  Product/1 -> Out1/1
  beta1/1 -> Pow/2

== system example1/ESTIMAT6/g11 ==
  x11 : Inport
  Sin : Trigonometry  Operator=cos
  g11 : Outport
  wires:
  Sin/1 -> g11/1
  x11/1 -> Sin/1

== system example1/ESTIMAT6/g12 ==
  x11 : Inport
  x12 : Inport  Port=2
  Add : Sum  Inputs=3
  Cos : Trigonometry  Operator=cos
  Gain : Gain  Gain=0.01
  Product : Product
  Sin : Trigonometry
  Sin1 : Trigonometry
  g12 : Outport
  wires:
  x12/1 -> Product/2, Sin/1
  Add/1 -> g12/1
  x11/1 -> Product/1, Cos/1
  Cos/1 -> Add/1
  Product/1 -> Gain/1
  Gain/1 -> Sin1/1
  Sin1/1 -> Add/3
  Sin/1 -> Add/2

== system example1/ESTIMAT7/[2]^1 ==
  In1 : Inport
  In2 : Inport  Port=2
  Abs : Abs  SaturateOnIntegerOverflow=off
  Pow : Math  Operator=pow  SignedPower=on  RndMeth=Zero
  Product : Product
  Sign : Signum
  Out1 : Outport
  wires:
  Pow/1 -> Product/1
  In2/1 -> Abs/1, Sign/1
  Abs/1 -> Pow/1
  Sign/1 -> Product/2
  Product/1 -> Out1/1
  In1/1 -> Pow/2

== system example1/ESTIMAT7/[2]^2 ==
  beta1 : Inport
  In2 : Inport  Port=2
  Abs : Abs  SaturateOnIntegerOverflow=off
  Pow : Math  Operator=pow  SignedPower=on  RndMeth=Zero
  Product : Product
  Sign : Signum
  Out1 : Outport
  wires:
  Pow/1 -> Product/1
  In2/1 -> Abs/1, Sign/1
  Abs/1 -> Pow/1
  Sign/1 -> Product/2
  Product/1 -> Out1/1
  beta1/1 -> Pow/2

== system example1/ESTIMAT7/[2]^3 ==
  In1 : Inport
  In2 : Inport  Port=2
  Abs : Abs  SaturateOnIntegerOverflow=off
  Pow : Math  Operator=pow  SignedPower=on  RndMeth=Zero
  Product : Product
  Sign : Signum
  Out1 : Outport
  wires:
  Pow/1 -> Product/1
  In2/1 -> Abs/1, Sign/1
  Abs/1 -> Pow/1
  Sign/1 -> Product/2
  Product/1 -> Out1/1
  In1/1 -> Pow/2

== system example1/ESTIMAT7/[2]^4 ==
  beta1 : Inport
  In2 : Inport  Port=2
  Abs : Abs  SaturateOnIntegerOverflow=off
  Pow : Math  Operator=pow  SignedPower=on  RndMeth=Zero
  Product : Product
  Sign : Signum
  Out1 : Outport
  wires:
  Pow/1 -> Product/1
  In2/1 -> Abs/1, Sign/1
  Abs/1 -> Pow/1
  Sign/1 -> Product/2
  Product/1 -> Out1/1
  beta1/1 -> Pow/2

== system example1/ESTIMAT7/[2]^5 ==
  In1 : Inport
  In2 : Inport  Port=2
  Abs : Abs  SaturateOnIntegerOverflow=off
  Pow : Math  Operator=pow  SignedPower=on  RndMeth=Zero
  Product : Product
  Sign : Signum
  Out1 : Outport
  wires:
  Pow/1 -> Product/1
  In2/1 -> Abs/1, Sign/1
  Abs/1 -> Pow/1
  Sign/1 -> Product/2
  Product/1 -> Out1/1
  In1/1 -> Pow/2

== system example1/ESTIMAT7/[2]^6 ==
  beta1 : Inport
  In2 : Inport  Port=2
  Abs : Abs  SaturateOnIntegerOverflow=off
  Pow : Math  Operator=pow  SignedPower=on  RndMeth=Zero
  Product : Product
  Sign : Signum
  Out1 : Outport
  wires:
  Pow/1 -> Product/1
  In2/1 -> Abs/1, Sign/1
  Abs/1 -> Pow/1
  Sign/1 -> Product/2
  Product/1 -> Out1/1
  beta1/1 -> Pow/2

== system example1/ESTIMAT7/g21 ==
  x21 : Inport
  Cos : Trigonometry  Operator=cos
  Product : Product
  Sin : Trigonometry
  g21 : Outport
  wires:
  x21/1 -> Cos/1, Sin/1
  Sin/1 -> Product/1
  Product/1 -> g21/1
  Cos/1 -> Product/2

== system example1/ESTIMAT7/g22 ==
  x21 : Inport
  x22 : Inport  Port=2
  Constant : Constant  Value=4/5
  Sin : Trigonometry
  Sum : Sum  Inputs=|++
  Sum1 : Sum  Inputs=|++
  "[2]^1_1" : Subsystem
  g22 : Outport
  wires:
  x22/1 -> "[2]^1_1"/2(2)
  Constant/1 -> "[2]^1_1"/1(In1)
  "[2]^1_1"/1(Out1) -> Sum/2
  Sum/1 -> g22/1
  x21/1 -> Sum1/1
  Sum1/1 -> Sin/1
  Sin/1 -> Sum/1

== system example1/ESTIMAT9/[2]^1 ==
  In1 : Inport
  In2 : Inport  Port=2
  Abs : Abs  SaturateOnIntegerOverflow=off
  Pow : Math  Operator=pow  SignedPower=on  RndMeth=Zero
  Product : Product
  Sign : Signum
  Out1 : Outport
  wires:
  Pow/1 -> Product/1
  In2/1 -> Abs/1, Sign/1
  Abs/1 -> Pow/1
  Sign/1 -> Product/2
  Product/1 -> Out1/1
  In1/1 -> Pow/2

== system example1/ESTIMAT9/[2]^2 ==
  beta1 : Inport
  In2 : Inport  Port=2
  Abs : Abs  SaturateOnIntegerOverflow=off
  Pow : Math  Operator=pow  SignedPower=on  RndMeth=Zero
  Product : Product
  Sign : Signum
  Out1 : Outport
  wires:
  Pow/1 -> Product/1
  In2/1 -> Abs/1, Sign/1
  Abs/1 -> Pow/1
  Sign/1 -> Product/2
  Product/1 -> Out1/1
  beta1/1 -> Pow/2

== system example1/ESTIMAT9/[2]^3 ==
  In1 : Inport
  In2 : Inport  Port=2
  Abs : Abs  SaturateOnIntegerOverflow=off
  Pow : Math  Operator=pow  SignedPower=on  RndMeth=Zero
  Product : Product
  Sign : Signum
  Out1 : Outport
  wires:
  Pow/1 -> Product/1
  In2/1 -> Abs/1, Sign/1
  Abs/1 -> Pow/1
  Sign/1 -> Product/2
  Product/1 -> Out1/1
  In1/1 -> Pow/2

== system example1/ESTIMAT9/[2]^4 ==
  beta1 : Inport
  In2 : Inport  Port=2
  Abs : Abs  SaturateOnIntegerOverflow=off
  Pow : Math  Operator=pow  SignedPower=on  RndMeth=Zero
  Product : Product
  Sign : Signum
  Out1 : Outport
  wires:
  Pow/1 -> Product/1
  In2/1 -> Abs/1, Sign/1
  Abs/1 -> Pow/1
  Sign/1 -> Product/2
  Product/1 -> Out1/1
  beta1/1 -> Pow/2

== system example1/ESTIMAT9/[2]^5 ==
  In1 : Inport
  In2 : Inport  Port=2
  Abs : Abs  SaturateOnIntegerOverflow=off
  Pow : Math  Operator=pow  SignedPower=on  RndMeth=Zero
  Product : Product
  Sign : Signum
  Out1 : Outport
  wires:
  Pow/1 -> Product/1
  In2/1 -> Abs/1, Sign/1
  Abs/1 -> Pow/1
  Sign/1 -> Product/2
  Product/1 -> Out1/1
  In1/1 -> Pow/2

== system example1/ESTIMAT9/[2]^6 ==
  beta1 : Inport
  In2 : Inport  Port=2
  Abs : Abs  SaturateOnIntegerOverflow=off
  Pow : Math  Operator=pow  SignedPower=on  RndMeth=Zero
  Product : Product
  Sign : Signum
  Out1 : Outport
  wires:
  Pow/1 -> Product/1
  In2/1 -> Abs/1, Sign/1
  Abs/1 -> Pow/1
  Sign/1 -> Product/2
  Product/1 -> Out1/1
  beta1/1 -> Pow/2

== system example1/ESTIMAT9/g1 ==
  x11 : Inport
  x12 : Inport  Port=2
  Cos : Trigonometry
  Sin : Trigonometry  Operator=cos
  Sum : Sum  Inputs=|++
  g12 : Outport
  wires:
  x12/1 -> Sin/1
  x11/1 -> Cos/1
  Cos/1 -> Sum/1
  Sin/1 -> Sum/2
  Sum/1 -> g12/1

== system example1/ESTIMAT9/g11 ==
  x11 : Inport
  Cos : Trigonometry
  Sum : Sum  Inputs=|++
  g11 : Outport
  wires:
  Cos/1 -> Sum/1
  Sum/1 -> g11/1
  x11/1 -> Sum/2, Cos/1

== system example1/SYSTEM1/f1 ==
  t : Inport
  x2 : Inport  Port=2
  x1 : Inport  Port=3
  Add : Sum  Inputs=5
  Constant : Constant  Value=2
  Gain : Gain  Gain=0.02
  Gain1 : Gain  Gain=0.01
  Sin : Trigonometry
  w : Trigonometry  Operator=cos
  f : Outport
  wires:
  Add/1 -> f/1
  x1/1 -> Gain1/1
  Sin/1 -> Add/2
  Constant/1 -> Add/4
  t/1 -> Gain/1
  w/1 -> Add/1
  Gain1/1 -> Sin/1
  Gain/1 -> w/1

== system example1/SYSTEM1/g11 ==
  x11 : Inport
  Cos : Trigonometry  Operator=cos
  Sum : Sum  Inputs=|++
  g11 : Outport
  wires:
  Cos/1 -> Sum/1
  Sum/1 -> g11/1
  x11/1 -> Sum/2, Cos/1

== system example1/SYSTEM1/g12 ==
  x11 : Inport
  x12 : Inport  Port=2
  Cos : Trigonometry  Operator=cos
  Sin : Trigonometry
  Sum : Sum  Inputs=|++
  g12 : Outport
  wires:
  x12/1 -> Sin/1
  x11/1 -> Cos/1
  Cos/1 -> Sum/1
  Sin/1 -> Sum/2
  Sum/1 -> g12/1

== system example1/SYSTEM2/f2 ==
  t : Inport
  x1 : Inport  Port=2
  Add : Sum  Inputs=3
  Cos : Trigonometry  Operator=cos
  Gain : Gain  Gain=0.1
  Gain1 : Gain  Gain=0.1
  Product : Product
  Sin : Trigonometry
  d2 : Constant  Value=3
  f2 : Outport
  wires:
  t/1 -> Gain1/1
  d2/1 -> Add/3
  Add/1 -> f2/1
  Product/1 -> Add/2
  Sin/1 -> Product/2
  x1/1 -> Gain/1
  Cos/1 -> Product/1
  Gain/1 -> Cos/1
  Gain1/1 -> Sin/1

== system example1/SYSTEM2/g21 ==
  x21 : Inport
  Cos : Trigonometry  Operator=cos
  Product : Product
  Sin : Trigonometry
  Sum : Sum  Inputs=|++
  g21 : Outport
  wires:
  x21/1 -> Cos/1, Sin/1, Sum/1
  Sum/1 -> g21/1
  Sin/1 -> Product/1
  Cos/1 -> Product/2
  Product/1 -> Sum/2

== system example1/SYSTEM2/g22 ==
  x21 : Inport
  x22 : Inport  Port=2
  Sin : Trigonometry
  Sum : Sum  Inputs=|++
  Sum1 : Sum  Inputs=|++
  g22 : Outport
  wires:
  x22/1 -> Sum/2, Sum1/2
  Sum/1 -> g22/1
  x21/1 -> Sum1/1
  Sum1/1 -> Sin/1
  Sin/1 -> Sum/1

== system example1/SYSTEM3/f1 ==
  t : Inport
  x1 : Inport  Port=2
  x2 : Inport  Port=3
  Add : Sum  Inputs=5
  Constant : Constant  Value=2
  Constant1 : Constant
  Cos : Trigonometry  Operator=cos
  Cos1 : Trigonometry
  Gain : Gain  Gain=0.01
  Gain1 : Gain  Gain=0.1
  Gain2 : Gain  Gain=0.01
  Product : Product
  w : Trigonometry  Operator=cos
  f : Outport
  wires:
  t/1 -> Gain/1
  Add/1 -> f/1
  x1/1 -> Product/1
  Product/1 -> Gain1/1
  Gain1/1 -> Cos/1
  w/1 -> Add/1
  Gain/1 -> w/1
  Cos/1 -> Add/2
  Constant1/1 -> Product/2
  x2/1 -> Gain2/1
  Gain2/1 -> Cos1/1
  Cos1/1 -> Add/3
  Constant/1 -> Add/5

== system example1/SYSTEM3/g11 ==
  x11 : Inport
  Sin : Trigonometry
  g11 : Outport
  wires:
  Sin/1 -> g11/1
  x11/1 -> Sin/1

== system example1/SYSTEM3/g12 ==
  x11 : Inport
  x12 : Inport  Port=2
  Add : Sum  Inputs=3
  Cos : Trigonometry  Operator=cos
  Product : Product
  Sin : Trigonometry
  Sin1 : Trigonometry
  g12 : Outport
  wires:
  x12/1 -> Product/2, Sin/1
  Sin/1 -> Add/2
  Add/1 -> g12/1
  x11/1 -> Product/1, Cos/1
  Cos/1 -> Add/1
  Product/1 -> Sin1/1

== system example1/SYSTEM4/f2 ==
  t : Inport
  x1 : Inport  Port=2
  x2 : Inport  Port=3
  Add : Sum  Inputs=3
  Cos : Trigonometry  Operator=cos
  Gain : Gain  Gain=0.05
  Gain1 : Gain  Gain=0.02
  Gain2 : Gain  Gain=0.5
  Sin : Trigonometry
  Sum : Sum  Inputs=|++
  d2 : Constant  Value=3
  f2 : Outport
  wires:
  Sin/1 -> Add/2
  d2/1 -> Add/3
  Add/1 -> f2/1
  Sum/1 -> Gain/1
  t/1 -> Sum/1
  x1/1 -> Sum/2
  x2/1 -> Gain1/1
  Cos/1 -> Gain2/1
  Gain/1 -> Sin/1
  Gain1/1 -> Cos/1
  Gain2/1 -> Add/1

== system example1/SYSTEM4/g21 ==
  x21 : Inport
  Cos : Trigonometry  Operator=cos
  Product : Product
  Product1 : Product
  Sin : Trigonometry
  g21 : Outport
  wires:
  x21/1 -> Cos/1, Sin/1
  Sin/1 -> Product/1
  Product/1 -> g21/1
  Cos/1 -> Product1/1, Product1/2
  Product1/1 -> Product/2

== system example1/SYSTEM4/g22 ==
  x21 : Inport
  x22 : Inport  Port=2
  Constant : Constant  Value=4/5
  Sin : Trigonometry
  Sum : Sum  Inputs=|++
  Sum1 : Sum  Inputs=|++
  "[2]^1_1" : Subsystem
  g22 : Outport
  wires:
  x22/1 -> Sum1/2, "[2]^1_1"/2(2)
  Constant/1 -> "[2]^1_1"/1(In1)
  "[2]^1_1"/1(Out1) -> Sum/2
  Sum/1 -> g22/1
  x21/1 -> Sum1/1
  Sum1/1 -> Sin/1
  Sin/1 -> Sum/1

== system example1/SYSTEM5/f1 ==
  t : Inport
  x2 : Inport  Port=2
  x1 : Inport  Port=3
  Add : Sum  Inputs=5
  Constant : Constant  Value=2
  Gain : Gain
  Gain1 : Gain  Gain=0.5
  Gain2 : Gain  Gain=0.05
  Sin : Trigonometry  Operator=cos
  w : Trigonometry  Operator=cos
  f : Outport
  wires:
  Add/1 -> f/1
  w/1 -> Gain/1
  x1/1 -> Gain1/1
  Sin/1 -> Add/2
  Constant/1 -> Add/4
  t/1 -> Gain2/1
  Gain/1 -> Add/1
  Gain1/1 -> Sin/1
  Gain2/1 -> w/1

== system example1/SYSTEM5/g11 ==
  x11 : Inport
  Cos : Trigonometry
  Sum : Sum  Inputs=|++
  g11 : Outport
  wires:
  Cos/1 -> Sum/1
  Sum/1 -> g11/1
  x11/1 -> Sum/2, Cos/1

== system example1/SYSTEM5/g12 ==
  x11 : Inport
  x12 : Inport  Port=2
  Cos : Trigonometry
  Sin : Trigonometry  Operator=cos
  Sum : Sum  Inputs=|++
  g12 : Outport
  wires:
  x12/1 -> Sin/1
  x11/1 -> Cos/1
  Cos/1 -> Sum/1
  Sin/1 -> Sum/2
  Sum/1 -> g12/1

== system example1/SYSTEM6/f2 ==
  t : Inport
  x1 : Inport  Port=2
  Add : Sum  Inputs=3
  Cos : Trigonometry  Operator=cos
  Gain : Gain  Gain=0.25
  Gain1 : Gain  Gain=0.05
  Product : Product
  Sin : Trigonometry
  d2 : Constant
  f2 : Outport
  wires:
  t/1 -> Gain1/1
  d2/1 -> Add/3
  Add/1 -> f2/1
  Product/1 -> Add/2
  Sin/1 -> Product/2
  Cos/1 -> Product/1
  x1/1 -> Gain/1
  Gain/1 -> Cos/1
  Gain1/1 -> Sin/1

== system example1/SYSTEM6/g21 ==
  x21 : Inport
  Cos : Trigonometry  Operator=cos
  Product : Product
  Sin : Trigonometry  Operator=cos
  Sum : Sum  Inputs=|++
  g21 : Outport
  wires:
  x21/1 -> Sum/1, Sin/1, Cos/1
  Sum/1 -> g21/1
  Sin/1 -> Product/1
  Cos/1 -> Product/2
  Product/1 -> Sum/2

== system example1/SYSTEM6/g22 ==
  x21 : Inport
  x22 : Inport  Port=2
  Gain : Gain  Gain=-2
  Sin : Trigonometry
  Sum : Sum  Inputs=|++
  Sum1 : Sum  Inputs=|++
  g22 : Outport
  wires:
  x22/1 -> Sum/2, Sum1/2
  Sum/1 -> g22/1
  x21/1 -> Gain/1
  Sum1/1 -> Sin/1
  Sin/1 -> Sum/1
  Gain/1 -> Sum1/1

== system example1/SYSTEM7/f1 ==
  t : Inport
  x1 : Inport  Port=2
  x2 : Inport  Port=3
  Add : Sum  Inputs=5
  Constant : Constant  Value=2
  Cos1 : Trigonometry  Operator=cos
  Gain : Gain  Gain=0.5
  Gain1 : Gain  Gain=0.05
  Gain2 : Gain  Gain=0.25
  Product1 : Product
  w : Trigonometry  Operator=cos
  f : Outport
  wires:
  t/1 -> Gain2/1
  Add/1 -> f/1
  w/1 -> Gain/1
  Constant/1 -> Add/5
  x1/1 -> Gain1/1
  Gain/1 -> Product1/2
  Product1/1 -> Add/1
  Cos1/1 -> Product1/1
  Gain1/1 -> Cos1/1
  Gain2/1 -> w/1

== system example1/SYSTEM7/g11 ==
  x11 : Inport
  Sin : Trigonometry  Operator=cos
  g11 : Outport
  wires:
  Sin/1 -> g11/1
  x11/1 -> Sin/1

== system example1/SYSTEM7/g12 ==
  x11 : Inport
  x12 : Inport  Port=2
  Add : Sum  Inputs=3
  Cos : Trigonometry  Operator=cos
  Gain : Gain  Gain=0.01
  Product : Product
  Sin : Trigonometry
  Sin1 : Trigonometry
  g12 : Outport
  wires:
  x12/1 -> Product/2, Sin/1
  Add/1 -> g12/1
  x11/1 -> Product/1, Cos/1
  Cos/1 -> Add/1
  Product/1 -> Gain/1
  Gain/1 -> Sin1/1
  Sin1/1 -> Add/3
  Sin/1 -> Add/2

== system example1/SYSTEM8/f2 ==
  t : Inport
  x1 : Inport  Port=2
  x2 : Inport  Port=3
  Add : Sum  Inputs=3
  Cos : Trigonometry  Operator=cos
  Gain : Gain  Gain=0.1
  Gain1 : Gain  Gain=0.25
  Sin : Trigonometry  Operator=cos
  Sum : Sum  Inputs=|++
  d2 : Constant  Value=2
  f2 : Outport
  wires:
  Sin/1 -> Add/2
  d2/1 -> Add/3
  Add/1 -> f2/1
  Sum/1 -> Gain/1
  t/1 -> Sum/1
  x1/1 -> Sum/2
  x2/1 -> Gain1/1
  Cos/1 -> Add/1
  Gain/1 -> Sin/1
  Gain1/1 -> Cos/1

== system example1/SYSTEM8/g21 ==
  x21 : Inport
  Cos : Trigonometry  Operator=cos
  Product : Product
  Sin : Trigonometry
  g21 : Outport
  wires:
  x21/1 -> Cos/1, Sin/1
  Sin/1 -> Product/1
  Product/1 -> g21/1
  Cos/1 -> Product/2

== system example1/SYSTEM8/g22 ==
  x21 : Inport
  x22 : Inport  Port=2
  Constant : Constant  Value=4/5
  Sin : Trigonometry
  Sum : Sum  Inputs=|++
  Sum1 : Sum  Inputs=|++
  "[2]^1_1" : Subsystem
  g22 : Outport
  wires:
  x22/1 -> "[2]^1_1"/2(2)
  Constant/1 -> "[2]^1_1"/1(In1)
  "[2]^1_1"/1(Out1) -> Sum/2
  Sum/1 -> g22/1
  x21/1 -> Sum1/1
  Sum1/1 -> Sin/1
  Sin/1 -> Sum/1

== system example1/Subsystem1/SAT ==
  In1 : Inport
  Constant : Constant  Value=-2000
  Constant1 : Constant  Value=2000
  If : If  IfExpression=u1 < -2000  ElseIfExpressions=u1 > 2000
  If Action Subsystem : Subsystem  TreatAsAtomicUnit=on
  If Action Subsystem1 : Subsystem  TreatAsAtomicUnit=on
  If Action Subsystem2 : Subsystem  TreatAsAtomicUnit=on
  Merge : Merge  Inputs=3
  u1 : Outport
  wires:
  In1/1 -> If Action Subsystem1/1(In1), If/1
  If/1 -> If Action Subsystem/Action
  Constant/1 -> If Action Subsystem/1(In1)
  If/3 -> If Action Subsystem1/Action
  If/2 -> If Action Subsystem2/Action
  Constant1/1 -> If Action Subsystem2/1(In1)
  If Action Subsystem/1(Out1) -> Merge/1
  If Action Subsystem1/1(Out1) -> Merge/3
  If Action Subsystem2/1(Out1) -> Merge/2
  Merge/1 -> u1/1

== system example1/Subsystem1/Subsystem ==
  alpha : Inport
  Abs : Abs  SaturateOnIntegerOverflow=off
  Abs1 : Abs  SaturateOnIntegerOverflow=off
  Add : Sum  Inputs=+-
  Constant : Constant  Value=1/2
  Constant1 : Constant  Value=2/3
  Divide : Product  Inputs=*/
  Gain : Gain  Gain=-1
  Integrator : Integrator
  Integrator1 : Integrator
  Pow : Math  Operator=pow  SignedPower=on  RndMeth=Zero
  Pow1 : Math  Operator=pow  SignedPower=on  RndMeth=Zero
  Product{,1..3} (4 alike) : Product
  Product4 : Product  Inputs=3
  Sign : Signum
  Sign1 : Signum
  Sum : Sum  Inputs=|++
  k1 : Constant  Value=0.01
  k2 : Constant  Value=0.1
  xi : Constant  Value=3
  tao1 : Outport
  tao2 : Outport  Port=2
  wires:
  alpha/1 -> Add/2
  Add/1 -> Pow/1, Sign/1
  Constant/1 -> Pow/2
  Pow/1 -> Abs/1
  Abs/1 -> Product/2
  Sign/1 -> Product/1
  Product/1 -> Product1/2
  k1/1 -> Product1/1
  Product1/1 -> Sum/1
  xi/1 -> Product4/2, Product4/3, Divide/2
  Divide/1 -> Sign1/1, Pow1/1
  Constant1/1 -> Pow1/2
  Pow1/1 -> Abs1/1
  Abs1/1 -> Product2/2
  Sign1/1 -> Product2/1
  Product2/1 -> Product3/1
  k2/1 -> Product3/2
  Product3/1 -> Sum/2
  Sum/1 -> Product4/1
  Product4/1 -> Gain/1
  Gain/1 -> Integrator/1
  Integrator/1 -> Divide/1, Integrator1/1, tao2/1
  Integrator1/1 -> Add/1, tao1/1

== system example1/Subsystem1/g1 ==
  x21 : Inport
  x22 : Inport  Port=2
  Gain : Gain  Gain=-2
  Sin : Trigonometry
  Sum : Sum  Inputs=|++
  Sum1 : Sum  Inputs=|++
  g22 : Outport
  wires:
  x22/1 -> Sum/2, Sum1/2
  Sum/1 -> g22/1
  x21/1 -> Gain/1
  Sum1/1 -> Sin/1
  Sin/1 -> Sum/1
  Gain/1 -> Sum1/1

== system example1/Subsystem10/SAT ==
  In1 : Inport
  Constant : Constant  Value=-1000
  Constant1 : Constant  Value=1000
  If : If  IfExpression=u1 < -1000  ElseIfExpressions=u1 > 1000
  If Action Subsystem : Subsystem  TreatAsAtomicUnit=on
  If Action Subsystem1 : Subsystem  TreatAsAtomicUnit=on
  If Action Subsystem2 : Subsystem  TreatAsAtomicUnit=on
  Merge : Merge  Inputs=3
  u1 : Outport
  wires:
  In1/1 -> If Action Subsystem1/1(In1), If/1
  If/1 -> If Action Subsystem/Action
  Constant/1 -> If Action Subsystem/1(In1)
  If/3 -> If Action Subsystem1/Action
  If/2 -> If Action Subsystem2/Action
  Constant1/1 -> If Action Subsystem2/1(In1)
  If Action Subsystem/1(Out1) -> Merge/1
  If Action Subsystem1/1(Out1) -> Merge/3
  If Action Subsystem2/1(Out1) -> Merge/2
  Merge/1 -> u1/1

== system example1/Subsystem10/Subsystem ==
  alpha : Inport
  Abs : Abs  SaturateOnIntegerOverflow=off
  Abs1 : Abs  SaturateOnIntegerOverflow=off
  Add : Sum  Inputs=+-
  Constant : Constant  Value=1/2
  Constant1 : Constant  Value=2/3
  Divide : Product  Inputs=*/
  Gain : Gain  Gain=-1
  Integrator : Integrator
  Integrator1 : Integrator
  Pow : Math  Operator=pow  SignedPower=on  RndMeth=Zero
  Pow1 : Math  Operator=pow  SignedPower=on  RndMeth=Zero
  Product{,1..3} (4 alike) : Product
  Product4 : Product  Inputs=3
  Sign : Signum
  Sign1 : Signum
  Sum : Sum  Inputs=|++
  k1 : Constant  Value=0.01
  k2 : Constant  Value=0.1
  xi : Constant
  tao1 : Outport
  tao2 : Outport  Port=2
  wires:
  alpha/1 -> Add/2
  Add/1 -> Pow/1, Sign/1
  Constant/1 -> Pow/2
  Pow/1 -> Abs/1
  Abs/1 -> Product/2
  Sign/1 -> Product/1
  Product/1 -> Product1/2
  k1/1 -> Product1/1
  Product1/1 -> Sum/1
  xi/1 -> Product4/2, Product4/3, Divide/2
  Divide/1 -> Sign1/1, Pow1/1
  Constant1/1 -> Pow1/2
  Pow1/1 -> Abs1/1
  Abs1/1 -> Product2/2
  Sign1/1 -> Product2/1
  Product2/1 -> Product3/1
  k2/1 -> Product3/2
  Product3/1 -> Sum/2
  Sum/1 -> Product4/1
  Product4/1 -> Gain/1
  Gain/1 -> Integrator/1
  Integrator/1 -> Divide/1, Integrator1/1, tao2/1
  Integrator1/1 -> Add/1, tao1/1

== system example1/Subsystem10/g22 ==
  x21 : Inport
  x22 : Inport  Port=2
  Sin : Trigonometry
  Sum : Sum  Inputs=|++
  Sum1 : Sum  Inputs=|++
  g22 : Outport
  wires:
  x22/1 -> Sum/2, Sum1/2
  Sum/1 -> g22/1
  x21/1 -> Sum1/1
  Sum1/1 -> Sin/1
  Sin/1 -> Sum/1

== system example1/Subsystem14/SAT ==
  In1 : Inport
  Constant : Constant  Value=-1000
  Constant1 : Constant  Value=1000
  If : If  IfExpression=u1 < -1000  ElseIfExpressions=u1 > 1000
  If Action Subsystem : Subsystem  TreatAsAtomicUnit=on
  If Action Subsystem1 : Subsystem  TreatAsAtomicUnit=on
  If Action Subsystem2 : Subsystem  TreatAsAtomicUnit=on
  Merge : Merge  Inputs=3
  u1 : Outport
  wires:
  In1/1 -> If Action Subsystem1/1(In1), If/1
  If/1 -> If Action Subsystem/Action
  Constant/1 -> If Action Subsystem/1(In1)
  If/3 -> If Action Subsystem1/Action
  If/2 -> If Action Subsystem2/Action
  Constant1/1 -> If Action Subsystem2/1(In1)
  If Action Subsystem/1(Out1) -> Merge/1
  If Action Subsystem1/1(Out1) -> Merge/3
  If Action Subsystem2/1(Out1) -> Merge/2
  Merge/1 -> u1/1

== system example1/Subsystem14/Subsystem ==
  alpha : Inport
  Abs : Abs  SaturateOnIntegerOverflow=off
  Abs1 : Abs  SaturateOnIntegerOverflow=off
  Add : Sum  Inputs=+-
  Constant : Constant  Value=1/2
  Constant1 : Constant  Value=2/3
  Divide : Product  Inputs=*/
  Gain : Gain  Gain=-1
  Integrator : Integrator
  Integrator1 : Integrator
  Pow : Math  Operator=pow  SignedPower=on  RndMeth=Zero
  Pow1 : Math  Operator=pow  SignedPower=on  RndMeth=Zero
  Product{,1..3} (4 alike) : Product
  Product4 : Product  Inputs=3
  Sign : Signum
  Sign1 : Signum
  Sum : Sum  Inputs=|++
  k1 : Constant  Value=0.01
  k2 : Constant  Value=0.1
  xi : Constant
  tao1 : Outport
  tao2 : Outport  Port=2
  wires:
  alpha/1 -> Add/2
  Add/1 -> Pow/1, Sign/1
  Constant/1 -> Pow/2
  Pow/1 -> Abs/1
  Abs/1 -> Product/2
  Sign/1 -> Product/1
  Product/1 -> Product1/2
  k1/1 -> Product1/1
  Product1/1 -> Sum/1
  xi/1 -> Product4/2, Product4/3, Divide/2
  Divide/1 -> Sign1/1, Pow1/1
  Constant1/1 -> Pow1/2
  Pow1/1 -> Abs1/1
  Abs1/1 -> Product2/2
  Sign1/1 -> Product2/1
  Product2/1 -> Product3/1
  k2/1 -> Product3/2
  Product3/1 -> Sum/2
  Sum/1 -> Product4/1
  Product4/1 -> Gain/1
  Gain/1 -> Integrator/1
  Integrator/1 -> Divide/1, Integrator1/1, tao2/1
  Integrator1/1 -> Add/1, tao1/1

== system example1/Subsystem14/[2]^1_1 ==
  p/q : Inport
  2 : Inport  Port=2
  Abs : Abs  SaturateOnIntegerOverflow=off
  Pow : Math  Operator=pow  SignedPower=on  RndMeth=Zero
  Product : Product
  Sign : Signum
  Out1 : Outport
  wires:
  2/1 -> Sign/1, Abs/1
  Abs/1 -> Pow/1
  p/q/1 -> Pow/2
  Pow/1 -> Product/2
  Sign/1 -> Product/1
  Product/1 -> Out1/1

== system example1/Subsystem14/[2]^1_2 ==
  In1 : Inport
  2 : Inport  Port=2
  Abs : Abs  SaturateOnIntegerOverflow=off
  Pow : Math  Operator=pow  SignedPower=on  RndMeth=Zero
  Product : Product
  Sign : Signum
  Out1 : Outport
  wires:
  2/1 -> Sign/1, Abs/1
  Abs/1 -> Pow/1
  In1/1 -> Pow/2
  Pow/1 -> Product/2
  Sign/1 -> Product/1
  Product/1 -> Out1/1

== system example1/Subsystem14/g12 ==
  x11 : Inport
  x12 : Inport  Port=2
  Add : Sum  Inputs=3
  Cos : Trigonometry  Operator=cos
  Product : Product
  Sin : Trigonometry
  Sin1 : Trigonometry
  g12 : Outport
  wires:
  x12/1 -> Product/2, Sin/1
  Sin/1 -> Add/2
  Add/1 -> g12/1
  x11/1 -> Product/1, Cos/1
  Cos/1 -> Add/1
  Product/1 -> Sin1/1
